simulink model "myControl"  (R2024b)
settings: Solver=VariableStepAuto  StartTime=0.0  StopTime=10.0  RelTol=1e-3
undefined symbols (not defined in the file): Kp, LedColor
settings Model: DataDictionary=myControlDictionary.sldd  Creator=rodri  LastModifiedBy=rodri

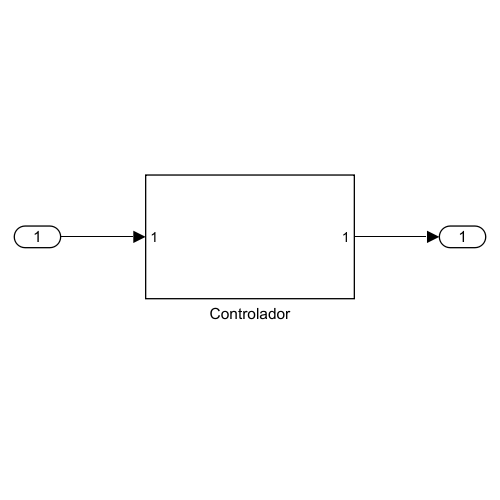
[thumbnail: Simulink's stored preview of the top-level diagram]
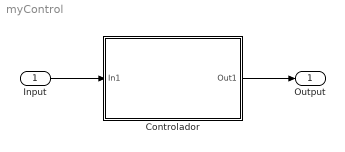
== system myControl ==
  Input : Inport
  Controlador : Subsystem
  Output : Outport
  wires:
  Input/1 -> Controlador/1(In1)
  Controlador/1(Out1) -> Output/1

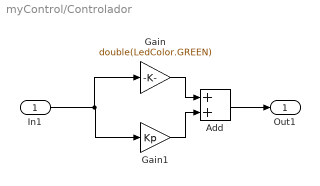
== system myControl/Controlador ==
  In1 : Inport
  Add : Sum
  Gain : Gain  Gain=double(LedColor.GREEN)
  Gain1 : Gain  Gain=Kp
  Out1 : Outport
  wires:
  In1/1 -> Gain/1, Gain1/1
  Gain/1 -> Add/1
  Gain1/1 -> Add/2
  Add/1 -> Out1/1
